simulink model "Pt_Transmission_CS9"  (Simulink 8.8)
settings: Solver=ode45  StartTime=0  StopTime=20  FixedStep=TSTEP  RelTol=1e-3  EnableMultiTasking=on
PreLoadFcn:
  | cd Extensions/Simulink/pt_transmission
  | mengine_carpet_eclass
  | torq_conv_map_eclass
  | Run_ft4wd_eclass
  | cd ../../..
undefined symbols (not defined in the file): ITC_OUTPUT_SHAFT, ITR, ITR_NEUTRAL, ITR_REVERSE, R_EFF_TR_F, R_EFF_TR_F_REVERSE, R_EFF_TR_R, R_EFF_TR_R_REVERSE, R_GEAR_TR, R_GEAR_TR_REVERSE
libraries: Solver_SF x1
settings Model: Creator=dhall  LastModifiedBy=mkhan  ExtModeTrigMode=oneshot  ExtModeArmWhenConnect=off
settings DataIOCC: LimitDataPoints=off  SaveOutput=off  SaveTime=off  SignalLoggingName=sigsOut
settings OptimizationCC: BooleanDataType=off  ExpressionDepthLimit=2147483647
settings DebuggingCC: SaveWithParameterizedLinksMsg=none  SignalResolutionControl=TryResolveAllWithWarning  MultiTaskDSMMsg=warning  MultiTaskCondExecSysMsg=none  SFExecutionAtInitializationDiag=warning
settings HardwareCC: TargetUnknown=on
settings GRTTargetCC: TargetFcnLib=ansi_tfl_tmw.mat  ModelReferenceCompliant=off  MatFileLogging=off
settings ConfigComp: CovSFcnEnable=off

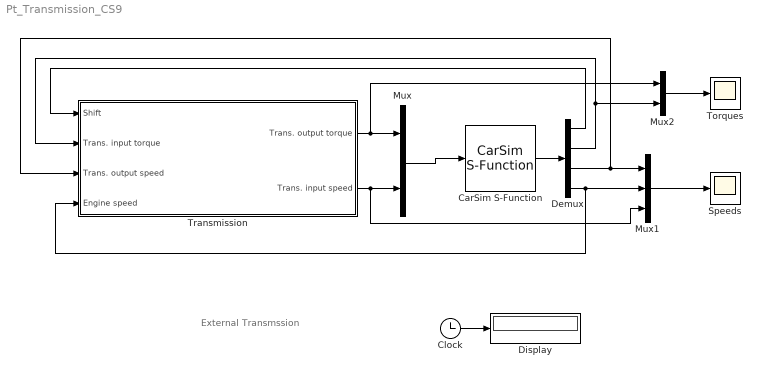
== system Pt_Transmission_CS9 ==
  note: External Transmssion
  CarSim S-Function : Solver_SF/CarSim S-Function  Priority=1  SIMFILE=simfile.sim  Run_RTs=off  vs_state_ind=Run  StopMode_ind=Vehicle Model
  Clock : Clock
  Demux : Demux
      settings: DisplayOption=none
  Display : Display
  Mux : Mux  Inputs=2
  Mux1 : Mux  Inputs=3
  Mux2 : Mux  Inputs=2
  Speeds : Scope
  Torques : Scope
  Transmission : Subsystem
  wires:
  Clock/1 -> Display/1
  Mux1/1 -> Speeds/1
  Transmission/1(Trans. output torque) -> Mux2/1, Mux/1
  Transmission/2(Trans. input speed) -> Mux/2, Mux1/3
  Demux/1 -> Transmission/1(Shift)
  Demux/2 -> Transmission/2(Trans. input torque), Mux2/2
  Demux/4 -> Mux1/2, Transmission/4(Engine speed)
  Demux/3 -> Transmission/3(Trans. output speed), Mux1/1
  Mux2/1 -> Torques/1
  CarSim S-Function/1 -> Demux/1
  Mux/1 -> CarSim S-Function/1

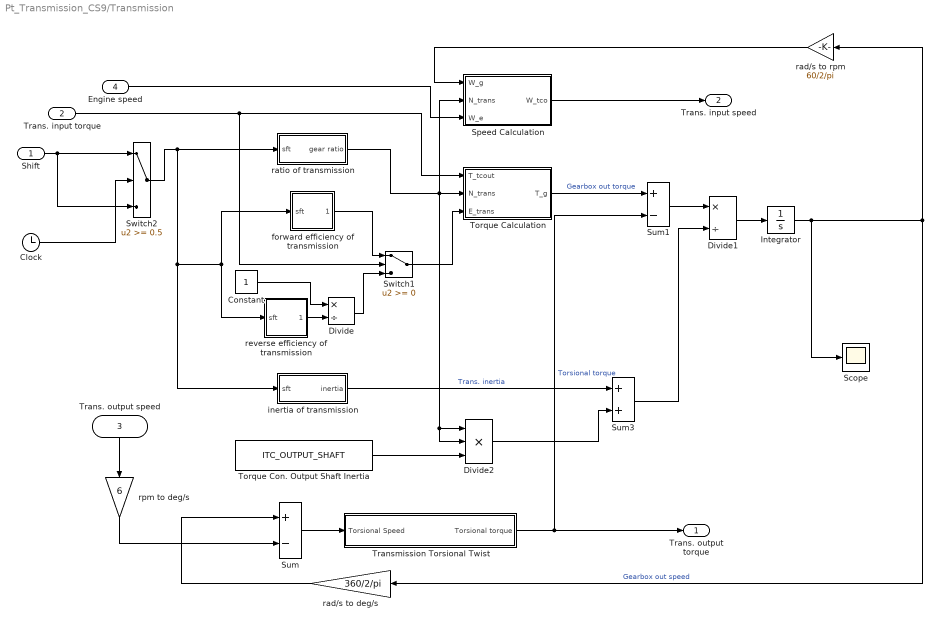
== system Pt_Transmission_CS9/Transmission ==
  Shift : Inport
  Trans. input torque : Inport  Port=2
  Trans. output speed : Inport  Port=3
  Engine speed : Inport  Port=4
  Clock : Clock
  Constant : Constant
  Divide : Product  Inputs=*/  InputSameDT=on  OutDataTypeStr=Inherit: Same as first input
  Divide1 : Product  Inputs=*/  InputSameDT=on  OutDataTypeStr=Inherit: Same as first input
  Divide2 : Product  Inputs=***  InputSameDT=on  OutDataTypeStr=Inherit: Same as first input
  Integrator : Integrator
  Scope : Scope
  Speed Calculation : Subsystem
  Sum : Sum  Inputs=+-  InputSameDT=on  SaturateOnIntegerOverflow=on  OutDataTypeStr=Inherit: Same as first input
  Sum1 : Sum  Inputs=+-  InputSameDT=on  SaturateOnIntegerOverflow=on  OutDataTypeStr=Inherit: Same as first input
  Sum3 : Sum  InputSameDT=on  SaturateOnIntegerOverflow=on  OutDataTypeStr=Inherit: Same as first input
  Switch1 : Switch  SaturateOnIntegerOverflow=on  InputSameDT=on
  Switch2 : Switch  Threshold=0.5  SaturateOnIntegerOverflow=on  InputSameDT=on
  Torque Calculation : Subsystem
  Torque Con. Output Shaft Inertia : Constant  Value=ITC_OUTPUT_SHAFT
  Transmission Torsional Twist : Subsystem
  forward efficiency of transmission : Subsystem  mask(forward efficiency of transmission){data=R_EFF_TR_F, data_rev=R_EFF_TR_F_REVERSE}
      mask prompts: data "gear"; data_rev "Reverse-gear"
  inertia of transmission : Subsystem  mask(forward efficiency of transmission){data=ITR, data_neu=ITR_NEUTRAL, data_rev=ITR_REVERSE}
      mask prompts: data "Inertia"; data_neu "Neutral inertia"; data_rev "Reverse-gear inertia"
      mask help:
      | input:
      |  sft is must be 0 - 7
      | output:
      |  transmission gear inertia
      | 1st parameta: inertia of forward gears
      | 2nd parameta: inertia of neutral
      | 3rd parameta: inertia of reverse gear
  rad/s to deg/s : Gain  Gain=360/2/pi  SaturateOnIntegerOverflow=on  OutDataTypeStr=Inherit: Same as input  ParamDataTypeStr=Inherit: Same as input
  rad/s to rpm : Gain  Gain=60/2/pi  SaturateOnIntegerOverflow=on  OutDataTypeStr=Inherit: Same as input  ParamDataTypeStr=Inherit: Same as input
  ratio of transmission : Subsystem  mask(forward efficiency of transmission){data=R_GEAR_TR, data_rev=R_GEAR_TR_REVERSE}
      mask prompts: data "gear ratio"; data_rev "Reverse-gear ratio"
      mask help:
      | input:
      |  sft is must be 0 - 7
      | output:
      |  transmission gear ratio
      |  when Nutral(0), it is zero
      | 1st parameta:
      |  must be vector
      | 2nd parameter:
      |  should be negative
  reverse efficiency of transmission : Subsystem  mask(reverse efficiency of transmission){data=R_EFF_TR_R, data_rev=R_EFF_TR_R_REVERSE}
      mask prompts: data "gear"; data_rev "Reverse-gear"
  rpm to deg/s : Gain  Gain=6  SaturateOnIntegerOverflow=on  OutDataTypeStr=Inherit: Same as input  ParamDataTypeStr=Inherit: Same as input
  Trans. output torque : Outport
  Trans. input speed : Outport  Port=2
  wires:
  Engine speed/1 -> Speed Calculation/3(W_e)
  forward efficiency of transmission/1(Out1) -> Switch1/1
  ratio of transmission/1(gear ratio) -> Torque Calculation/2(N_trans), Speed Calculation/2(N_trans), Divide2/1, Divide2/2
  Trans. input torque/1 -> Torque Calculation/1(T_tcout), Switch1/2
  Switch1/1 -> Torque Calculation/3(E_trans)
  Speed Calculation/1(W_tco) -> Trans. input speed/1
  Switch2/1 -> ratio of transmission/1(sft), reverse efficiency of transmission/1(sft), forward efficiency of transmission/1(sft), inertia of transmission/1(sft)
  Clock/1 -> Switch2/2
  Shift/1 -> Switch2/1, Switch2/3
  reverse efficiency of transmission/1(Out1) -> Divide/2
  Divide/1 -> Switch1/3
  Constant/1 -> Divide/1
  Torque Calculation/1(T_g) -> Sum1/1  "Gearbox out torque"
  Trans. output speed/1 -> rpm to deg/s/1
  rpm to deg/s/1 -> Sum/2
  Sum/1 -> Transmission Torsional Twist/1(Torsional Speed)
  Transmission Torsional Twist/1(Torsional torque) -> Sum1/2, Trans. output torque/1  "Torsional torque"
  Divide1/1 -> Integrator/1
  Integrator/1 -> rad/s to rpm/1, rad/s to deg/s/1, Scope/1  "Gearbox out speed"
  Sum1/1 -> Divide1/1
  inertia of transmission/1(inertia) -> Sum3/1  "Trans. inertia"
  Sum3/1 -> Divide1/2
  rad/s to rpm/1 -> Speed Calculation/1(W_g)
  Torque Con. Output Shaft Inertia/1 -> Divide2/3
  Divide2/1 -> Sum3/2
  rad/s to deg/s/1 -> Sum/1

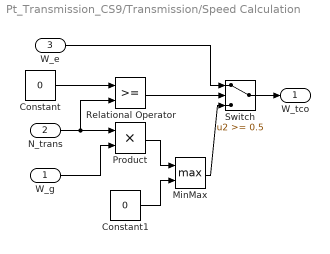
== system Pt_Transmission_CS9/Transmission/Speed Calculation ==
  W_g : Inport
  N_trans : Inport  Port=2
  W_e : Inport  Port=3
  Constant : Constant  Value=0
  Constant1 : Constant  Value=0
  MinMax : MinMax  Function=max  Inputs=2  InputSameDT=on  SaturateOnIntegerOverflow=on
  Product : Product  InputSameDT=on  SaturateOnIntegerOverflow=on  OutDataTypeStr=Inherit: Same as first input
  Relational Operator : RelationalOperator  RndMeth=Nearest  InputSameDT=on
  Switch : Switch  Threshold=0.5  SaturateOnIntegerOverflow=on  InputSameDT=on
  W_tco : Outport
  wires:
  MinMax/1 -> Switch/3
  Product/1 -> MinMax/1
  Constant1/1 -> MinMax/2
  Switch/1 -> W_tco/1
  N_trans/1 -> Relational Operator/2, Product/1
  Constant/1 -> Relational Operator/1
  W_e/1 -> Switch/1
  Relational Operator/1 -> Switch/2
  W_g/1 -> Product/2

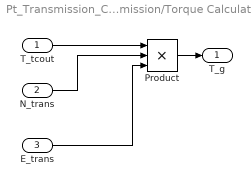
== system Pt_Transmission_CS9/Transmission/Torque Calculation ==
  T_tcout : Inport
  N_trans : Inport  Port=2
  E_trans : Inport  Port=3
  Product : Product  Inputs=3  InputSameDT=on  SaturateOnIntegerOverflow=on  OutDataTypeStr=Inherit: Same as first input
  T_g : Outport
  wires:
  N_trans/1 -> Product/2
  T_tcout/1 -> Product/1
  E_trans/1 -> Product/3
  Product/1 -> T_g/1

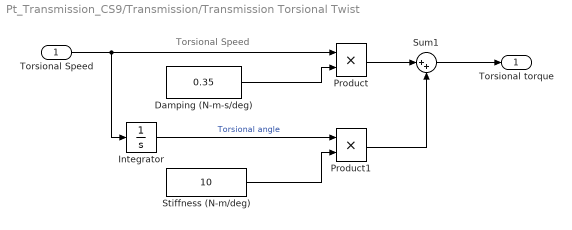
== system Pt_Transmission_CS9/Transmission/Transmission Torsional Twist ==
  note: Torsional Speed
  Torsional Speed : Inport
  Damping (N-m-s/deg) : Constant  Value=0.35
  Integrator : Integrator
  Product : Product  InputSameDT=on  SaturateOnIntegerOverflow=on  OutDataTypeStr=Inherit: Same as first input
  Product1 : Product  InputSameDT=on  SaturateOnIntegerOverflow=on  OutDataTypeStr=Inherit: Same as first input
  Stiffness (N-m/deg) : Constant  Value=10
  Sum1 : Sum  Inputs=|++  InputSameDT=on  SaturateOnIntegerOverflow=on  OutDataTypeStr=Inherit: Same as first input
  Torsional torque : Outport
  wires:
  Stiffness (N-m/deg)/1 -> Product1/2
  Damping (N-m-s/deg)/1 -> Product/2
  Product/1 -> Sum1/1
  Product1/1 -> Sum1/2
  Sum1/1 -> Torsional torque/1
  Torsional Speed/1 -> Product/1, Integrator/1
  Integrator/1 -> Product1/1  "Torsional angle"

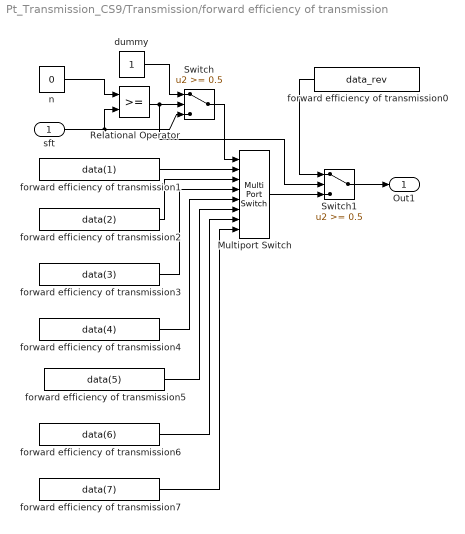
== system Pt_Transmission_CS9/Transmission/forward efficiency of transmission ==
  sft : Inport
  Multiport Switch : MultiPortSwitch  Inputs=7  SaturateOnIntegerOverflow=on  InputSameDT=on
  Relational Operator : RelationalOperator  RndMeth=Nearest  InputSameDT=on
  Switch : Switch  Threshold=0.5  SaturateOnIntegerOverflow=on  InputSameDT=on
  Switch1 : Switch  Threshold=0.5  SaturateOnIntegerOverflow=on  InputSameDT=on
  dummy : Constant
  forward efficiency of transmission0 : Constant  Value=data_rev
  forward efficiency of transmission1 : Constant  Value=data(1)
  forward efficiency of transmission2 : Constant  Value=data(2)
  forward efficiency of transmission3 : Constant  Value=data(3)
  forward efficiency of transmission4 : Constant  Value=data(4)
  forward efficiency of transmission5 : Constant  Value=data(5)
  forward efficiency of transmission6 : Constant  Value=data(6)
  forward efficiency of transmission7 : Constant  Value=data(7)
  n : Constant  Value=0
  Out1 : Outport
  wires:
  dummy/1 -> Switch/1
  forward efficiency of transmission0/1 -> Switch1/1
  Relational Operator/1 -> Switch1/2, Switch/2
  n/1 -> Relational Operator/1
  sft/1 -> Switch/3, Relational Operator/2
  Multiport Switch/1 -> Switch1/3
  Switch1/1 -> Out1/1
  forward efficiency of transmission7/1 -> Multiport Switch/8
  forward efficiency of transmission6/1 -> Multiport Switch/7
  forward efficiency of transmission5/1 -> Multiport Switch/6
  forward efficiency of transmission4/1 -> Multiport Switch/5
  forward efficiency of transmission3/1 -> Multiport Switch/4
  forward efficiency of transmission2/1 -> Multiport Switch/3
  Switch/1 -> Multiport Switch/1
  forward efficiency of transmission1/1 -> Multiport Switch/2

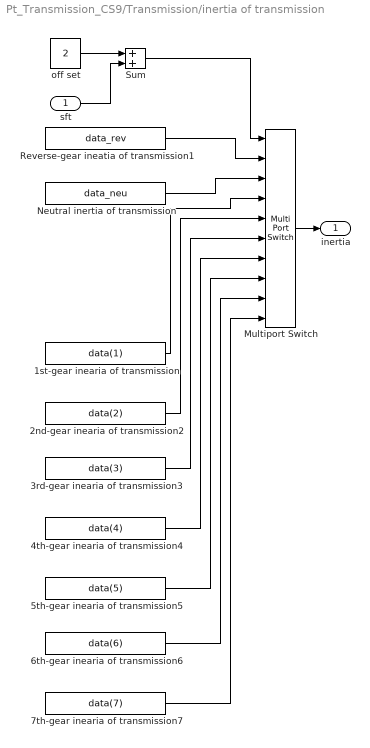
== system Pt_Transmission_CS9/Transmission/inertia of transmission ==
  sft : Inport
  1st-gear inearia of transmission : Constant  Value=data(1)
  2nd-gear inearia of transmission2 : Constant  Value=data(2)
  3rd-gear inearia of transmission3 : Constant  Value=data(3)
  4th-gear inearia of transmission4 : Constant  Value=data(4)
  5th-gear inearia of transmission5 : Constant  Value=data(5)
  6th-gear inearia of transmission6 : Constant  Value=data(6)
  7th-gear inearia of transmission7 : Constant  Value=data(7)
  Multiport Switch : MultiPortSwitch  Inputs=9  SaturateOnIntegerOverflow=on  InputSameDT=on
  Neutral inertia of transmission : Constant  Value=data_neu
  Reverse-gear ineatia of transmission1 : Constant  Value=data_rev
  Sum : Sum  Inputs=2  InputSameDT=on  SaturateOnIntegerOverflow=on  OutDataTypeStr=Inherit: Same as first input
  off set : Constant  Value=2
  inertia : Outport
  wires:
  Neutral inertia of transmission/1 -> Multiport Switch/3
  Sum/1 -> Multiport Switch/1
  Reverse-gear ineatia of transmission1/1 -> Multiport Switch/2
  7th-gear inearia of transmission7/1 -> Multiport Switch/10
  6th-gear inearia of transmission6/1 -> Multiport Switch/9
  5th-gear inearia of transmission5/1 -> Multiport Switch/8
  4th-gear inearia of transmission4/1 -> Multiport Switch/7
  3rd-gear inearia of transmission3/1 -> Multiport Switch/6
  2nd-gear inearia of transmission2/1 -> Multiport Switch/5
  1st-gear inearia of transmission/1 -> Multiport Switch/4
  Multiport Switch/1 -> inertia/1
  off set/1 -> Sum/1
  sft/1 -> Sum/2

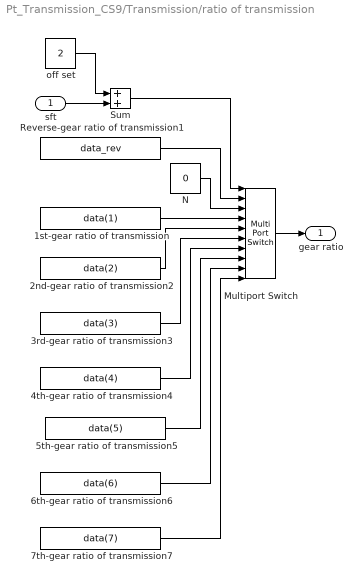
== system Pt_Transmission_CS9/Transmission/ratio of transmission ==
  sft : Inport
  1st-gear ratio of transmission : Constant  Value=data(1)
  2nd-gear ratio of transmission2 : Constant  Value=data(2)
  3rd-gear ratio of transmission3 : Constant  Value=data(3)
  4th-gear ratio of transmission4 : Constant  Value=data(4)
  5th-gear ratio of transmission5 : Constant  Value=data(5)
  6th-gear ratio of transmission6 : Constant  Value=data(6)
  7th-gear ratio of transmission7 : Constant  Value=data(7)
  Multiport Switch : MultiPortSwitch  Inputs=9  SaturateOnIntegerOverflow=on  InputSameDT=on
  N : Constant  Value=0
  Reverse-gear ratio of transmission1 : Constant  Value=data_rev
  Sum : Sum  Inputs=2  InputSameDT=on  SaturateOnIntegerOverflow=on  OutDataTypeStr=Inherit: Same as first input
  off set : Constant  Value=2
  gear ratio : Outport
  wires:
  N/1 -> Multiport Switch/3
  Sum/1 -> Multiport Switch/1
  Reverse-gear ratio of transmission1/1 -> Multiport Switch/2
  7th-gear ratio of transmission7/1 -> Multiport Switch/10
  6th-gear ratio of transmission6/1 -> Multiport Switch/9
  5th-gear ratio of transmission5/1 -> Multiport Switch/8
  4th-gear ratio of transmission4/1 -> Multiport Switch/7
  3rd-gear ratio of transmission3/1 -> Multiport Switch/6
  2nd-gear ratio of transmission2/1 -> Multiport Switch/5
  1st-gear ratio of transmission/1 -> Multiport Switch/4
  Multiport Switch/1 -> gear ratio/1
  off set/1 -> Sum/1
  sft/1 -> Sum/2

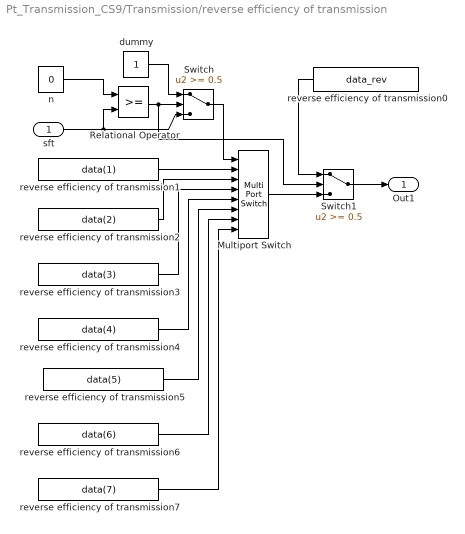
== system Pt_Transmission_CS9/Transmission/reverse efficiency of transmission ==
  sft : Inport
  Multiport Switch : MultiPortSwitch  Inputs=7  SaturateOnIntegerOverflow=on  InputSameDT=on
  Relational Operator : RelationalOperator  RndMeth=Nearest  InputSameDT=on
  Switch : Switch  Threshold=0.5  SaturateOnIntegerOverflow=on  InputSameDT=on
  Switch1 : Switch  Threshold=0.5  SaturateOnIntegerOverflow=on  InputSameDT=on
  dummy : Constant
  n : Constant  Value=0
  reverse efficiency of transmission0 : Constant  Value=data_rev
  reverse efficiency of transmission1 : Constant  Value=data(1)
  reverse efficiency of transmission2 : Constant  Value=data(2)
  reverse efficiency of transmission3 : Constant  Value=data(3)
  reverse efficiency of transmission4 : Constant  Value=data(4)
  reverse efficiency of transmission5 : Constant  Value=data(5)
  reverse efficiency of transmission6 : Constant  Value=data(6)
  reverse efficiency of transmission7 : Constant  Value=data(7)
  Out1 : Outport
  wires:
  dummy/1 -> Switch/1
  reverse efficiency of transmission0/1 -> Switch1/1
  reverse efficiency of transmission1/1 -> Multiport Switch/2
  Switch/1 -> Multiport Switch/1
  reverse efficiency of transmission2/1 -> Multiport Switch/3
  reverse efficiency of transmission3/1 -> Multiport Switch/4
  reverse efficiency of transmission4/1 -> Multiport Switch/5
  reverse efficiency of transmission5/1 -> Multiport Switch/6
  reverse efficiency of transmission6/1 -> Multiport Switch/7
  reverse efficiency of transmission7/1 -> Multiport Switch/8
  Switch1/1 -> Out1/1
  Multiport Switch/1 -> Switch1/3
  sft/1 -> Relational Operator/2, Switch/3
  n/1 -> Relational Operator/1
  Relational Operator/1 -> Switch/2, Switch1/2
